simulink model "Lyp1"  (R2018b)
settings: Solver=FixedStepAuto  StartTime=0.0  StopTime=10.0  FixedStep=0.001  RelTol=1e-3  EnableMultiTasking=on
InitFcn:
  | X0 = randn(1)*10 ;
settings Model: Creator=omid_zandi  LastModifiedBy=Arash
settings OptimizationCC: LifeSpan=inf
settings DebuggingCC: SFUnexpectedBacktrackingDiag=warning  SFNoUnconditionalDefaultTransitionDiag=warning
settings SFSimCC: SimUseLocalCustomCode=off
settings RTWCC: RTWUseLocalCustomCode=off
settings CodeAppCC: StateflowObjectComments=on
settings GRTTargetCC: TargetLangStandard=C89/C90 (ANSI)  GeneratePreprocessorConditionals=Disable all
settings ConfigComp: CovMetricSettings=dw  CovHtmlReporting=on  CovSaveCumulativeToWorkspaceVar=on  CovSaveSingleToWorkspaceVar=on  CovExternalEMLEnable=off

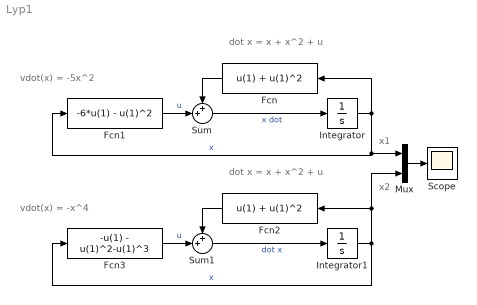
== system Lyp1 ==
  note: x2
  note: x1
  note: vdot(x) = -x^4
  note: vdot(x) = -5x^2
  note: dot x = x + x^2 + u
  note: dot x = x + x^2 + u
  Fcn : Fcn  Expr=u(1) + u(1)^2
  Fcn1 : Fcn  Expr=-6*u(1) - u(1)^2
  Fcn2 : Fcn  Expr=u(1) + u(1)^2
  Fcn3 : Fcn  Expr=-u(1) - u(1)^2-u(1)^3
  Integrator : Integrator  InitialCondition=X0
  Integrator1 : Integrator  InitialCondition=X0
  Mux : Mux  Inputs=2
  Scope : Scope
  Sum : Sum  Inputs=++|
  Sum1 : Sum  Inputs=++|
  wires:
  Integrator/1 -> Fcn1/1, Mux/1, Fcn/1  "x"
  Sum/1 -> Integrator/1  "x dot"
  Fcn/1 -> Sum/1
  Fcn1/1 -> Sum/2  "u"
  Integrator1/1 -> Mux/2, Fcn2/1, Fcn3/1  "x"
  Sum1/1 -> Integrator1/1  "dot x"
  Fcn2/1 -> Sum1/1
  Fcn3/1 -> Sum1/2  "u"
  Mux/1 -> Scope/1
